simulink model "modele17"  (R2019a)
settings: Solver=VariableStepAuto  StartTime=0.0  StopTime=1  RelTol=1e-4
values from neighbouring files (symbols this model uses):
  Cb = 9.97*(10^(-2))    (= 0.0997)    [parametres_cubli.m]
  Cw = 2.95e-5    (= 2.95e-05)    [parametres_cubli.m]
  g = 9.81    [parametres_cubli.m]
  Ib = 3.43*(10^(-3))    (= 0.00343)    [parametres_cubli.m]
  Iw = 2.63*(10^(-4))    (= 0.000263)    [parametres_cubli.m]
  l = 9.65*0.01    (= 0.0965)    [parametres_cubli.m]
  lb = 10.35*0.01    (= 0.1035)    [parametres_cubli.m]
  mb = 0.43    [parametres_cubli.m]
  mw = 0.096    [parametres_cubli.m]
  Theta_b_ini = 0.125    [parametres_cubli.m]
  Tm_sat = 3.0    (= 3)    [parametres_cubli.m]
undefined symbols (not defined in the file or in its folder): K3, sigbuilder_block
settings Model: Creator=ntest557  LastModifiedBy=ntest
settings SolverCC: ZeroCrossAlgorithm=Adaptive
settings DataIOCC: ReturnWorkspaceOutputs=off
settings DebuggingCC: IgnoredZcDiagnostic=none  ArithmeticOperatorsInVariantConditions=warning
settings CodeAppCC: StateflowObjectComments=on

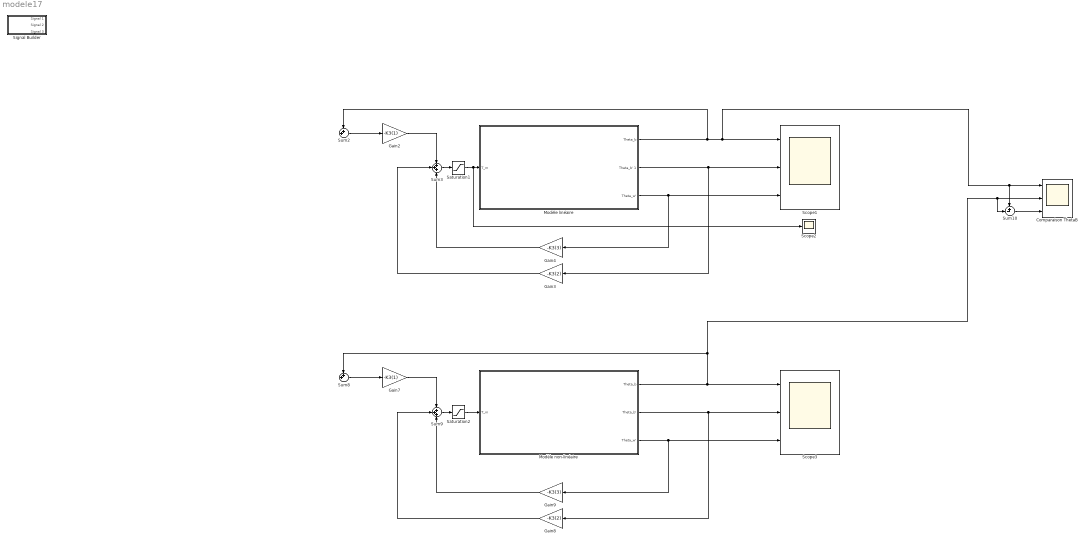
== system modele17 ==
  "Comparaison ThetaB " : Scope  NumInputPorts=3
  Gain2 : Gain  Gain=-K3(1)
  Gain3 : Gain  Gain=-K3(2)
  Gain4 : Gain  Gain=-K3(3)
  Gain7 : Gain  Gain=-K3(1)
  Gain8 : Gain  Gain=-K3(2)
  Gain9 : Gain  Gain=-K3(3)
  Modèle linéaire : Subsystem
  "Modèle non-linéaire " : Subsystem
  Saturation1 : Saturate  UpperLimit=Tm_sat  LowerLimit=-Tm_sat
  Saturation2 : Saturate  UpperLimit=Tm_sat  LowerLimit=-Tm_sat
  Scope1 : Scope  NumInputPorts=3
  Scope2 : Scope
  Scope3 : Scope  NumInputPorts=3
  Signal Builder : Subsystem  Tag=STV Subsys  LoadFcn=sigbuilder_block('load');  StartFcn=sigbuilder_block('start');  StopFcn=sigbuilder_block('stop');  ClipboardFcn=sigbuilder_block('clipboard');  mask(Sigbuilder block){tuvar=[0:10]}
      mask help: Simulink:masks:SigbuilderBlock_MD
      mask init:
      | if ~strcmp(get_param(bdroot(gcbh),'SimulationStatus'),'stopped') tuvar = sigbuilder_block('maskInit'); end
      settings: CopyFcn=sigbuilder_block('copy');  DeleteFcn=sigbuilder_block('delete');  ModelCloseFcn=sigbuilder_block('modelClose');  PreSaveFcn=sigbuilder_block('preSave');  PauseFcn=sigbuilder_block('pause');  ContinueFcn=sigbuilder_block('continue');  NameChangeFcn=sigbuilder_block('namechange');  OpenFcn=sigbuilder_block('open',[6 30 1248 660 ]);  CloseFcn=sigbuilder_block('close');
      mask Display: plot(0, 0, 100, 100,[2, 2, 32, 32, 2], [68, 8, 8, 68, 68],[32, 2], [38, 38], [32, 19, 2],[53, 60, 44], [32, 17, 17, 2],[16, 16, 31, 31]);txt = getActiveGroup(gcbh);text(2, 100, txt,'verticalAlignment', 'top');
  Sum10 : Sum  Inputs=+-|
  Sum2 : Sum  Inputs=++|
  Sum3 : Sum  Inputs=+++
  Sum8 : Sum  Inputs=++|
  Sum9 : Sum  Inputs=+++
  wires:
  "Modèle non-linéaire "/1("Theta_b ") -> Scope3/1, Sum10/2, "Comparaison ThetaB "/2, Sum8/1
  "Modèle non-linéaire "/2("Theta_b' ") -> Scope3/2, Gain8/1
  "Modèle non-linéaire "/3(Theta_w') -> Scope3/3, Gain9/1
  Sum8/1 -> Gain7/1
  Gain7/1 -> Sum9/1
  Gain8/1 -> Sum9/2
  Gain9/1 -> Sum9/3
  Sum10/1 -> "Comparaison ThetaB "/3
  Gain4/1 -> Sum3/3
  Gain3/1 -> Sum3/2
  Sum2/1 -> Gain2/1
  Gain2/1 -> Sum3/1
  Modèle linéaire/3(Theta_w') -> Scope1/3, Gain4/1
  Saturation1/1 -> Modèle linéaire/1("T_m "), Scope2/1
  Modèle linéaire/1("Theta_b ") -> Sum2/1, Sum10/1, "Comparaison ThetaB "/1, Scope1/1
  Modèle linéaire/2(Theta_b' 1) -> Gain3/1, Scope1/2
  Sum3/1 -> Saturation1/1
  Sum9/1 -> Saturation2/1
  Saturation2/1 -> "Modèle non-linéaire "/1("T_m ")

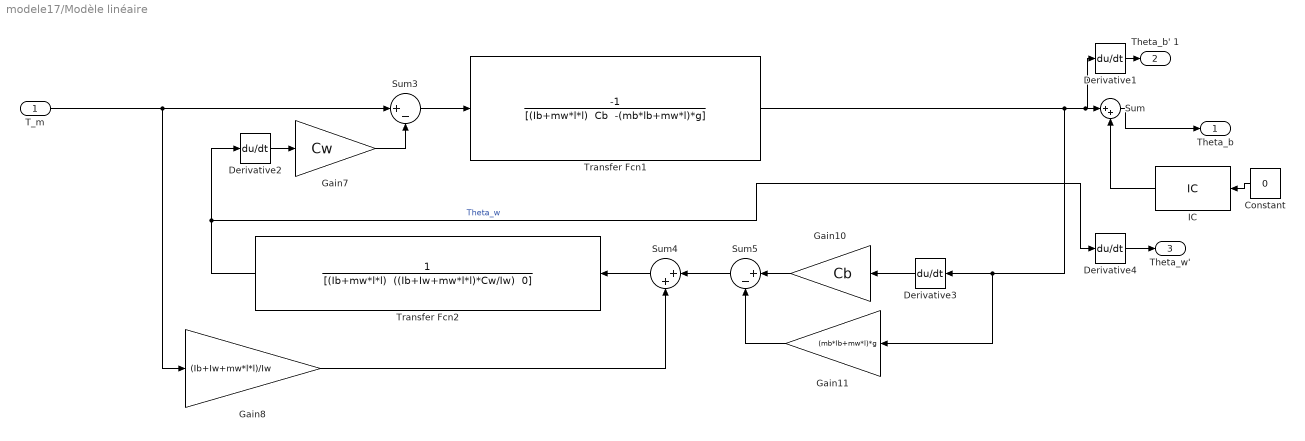
== system modele17/Modèle linéaire ==
  "T_m " : Inport
  Constant : Constant  Value=0
  Derivative{1..4} (4 alike) : Derivative
  Gain10 : Gain  Gain=Cb
  Gain11 : Gain  Gain=(mb*lb+mw*l)*g
  Gain7 : Gain  Gain=Cw
  Gain8 : Gain  Gain=(Ib+Iw+mw*l*l)/Iw
  IC : InitialCondition  Value=Theta_b_ini
  Sum : Sum  Inputs=|++
  Sum3 : Sum  Inputs=|+-
  Sum4 : Sum  Inputs=|++
  Sum5 : Sum  Inputs=|+-
  Transfer Fcn1 : TransferFcn  Numerator=[-1]  Denominator="[(Ib+mw*l*l)  Cb  -(mb*lb+mw*l)*g]"  ContinuousStateAttributes="\"Theta_b_ini\""
  Transfer Fcn2 : TransferFcn  Denominator="[(Ib+mw*l*l)  ((Ib+Iw+mw*l*l)*Cw/Iw)  0]"
  "Theta_b " : Outport
  Theta_b' 1 : Outport  Port=2
  Theta_w' : Outport  Port=3
  wires:
  Transfer Fcn2/1 -> Derivative4/1, Derivative2/1  "Theta_w"
  Gain8/1 -> Sum4/2
  Sum4/1 -> Transfer Fcn2/1
  "T_m "/1 -> Gain8/1, Sum3/1
  Gain10/1 -> Sum5/1
  Derivative2/1 -> Gain7/1
  Sum3/1 -> Transfer Fcn1/1
  Gain7/1 -> Sum3/2
  Derivative3/1 -> Gain10/1
  Sum5/1 -> Sum4/1
  Gain11/1 -> Sum5/2
  Derivative4/1 -> Theta_w'/1
  Derivative1/1 -> Theta_b' 1/1
  Transfer Fcn1/1 -> Derivative3/1, Gain11/1, Derivative1/1, Sum/1
  Sum/1 -> "Theta_b "/1
  Constant/1 -> IC/1
  IC/1 -> Sum/2

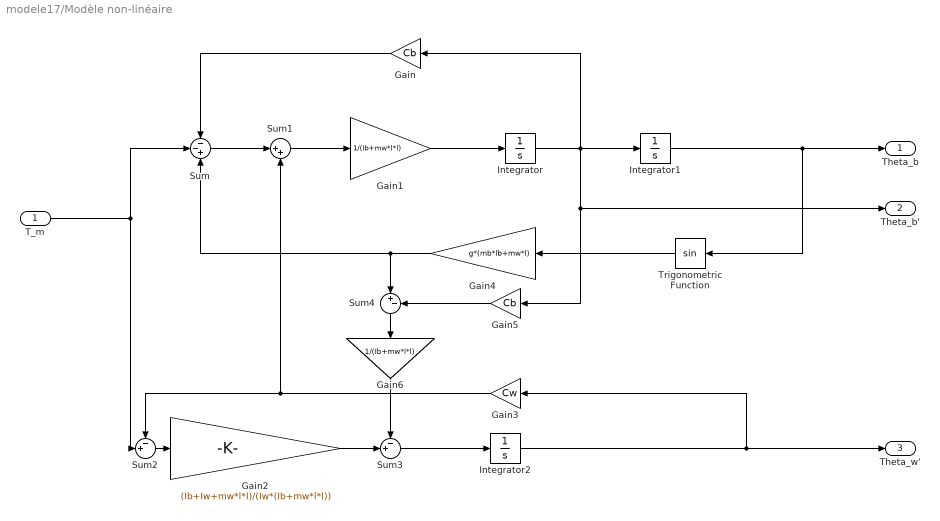
== system modele17/Modèle non-linéaire  ==
  "T_m " : Inport
  Gain : Gain  Gain=Cb
  Gain1 : Gain  Gain=1/(Ib+mw*l*l)
  Gain2 : Gain  Gain=(Ib+Iw+mw*l*l)/(Iw*(Ib+mw*l*l))
  Gain3 : Gain  Gain=Cw
  Gain4 : Gain  Gain=g*(mb*lb+mw*l)
  Gain5 : Gain  Gain=Cb
  Gain6 : Gain  Gain=1/(Ib+mw*l*l)
  Integrator : Integrator
  Integrator1 : Integrator  InitialCondition=Theta_b_ini
  Integrator2 : Integrator
  Sum : Sum  Inputs=--+
  Sum1 : Sum  Inputs=|++
  Sum2 : Sum  Inputs=-+|
  Sum3 : Sum  Inputs=-+|
  Sum4 : Sum  Inputs=|+-
  Trigonometric Function : Trigonometry
  "Theta_b " : Outport
  "Theta_b' " : Outport  Port=2
  Theta_w' : Outport  Port=3
  wires:
  Gain/1 -> Sum/1
  Sum/1 -> Sum1/1
  Sum1/1 -> Gain1/1
  Gain1/1 -> Integrator/1
  Integrator/1 -> "Theta_b' "/1, Gain5/1, Gain/1, Integrator1/1
  "T_m "/1 -> Sum/2, Sum2/2
  Integrator1/1 -> Trigonometric Function/1, "Theta_b "/1
  Sum2/1 -> Gain2/1
  Gain2/1 -> Sum3/2
  Sum3/1 -> Integrator2/1
  Integrator2/1 -> Gain3/1, Theta_w'/1
  Gain3/1 -> Sum1/2, Sum2/1
  Trigonometric Function/1 -> Gain4/1
  Gain4/1 -> Sum/3, Sum4/1
  Sum4/1 -> Gain6/1
  Gain5/1 -> Sum4/2
  Gain6/1 -> Sum3/1

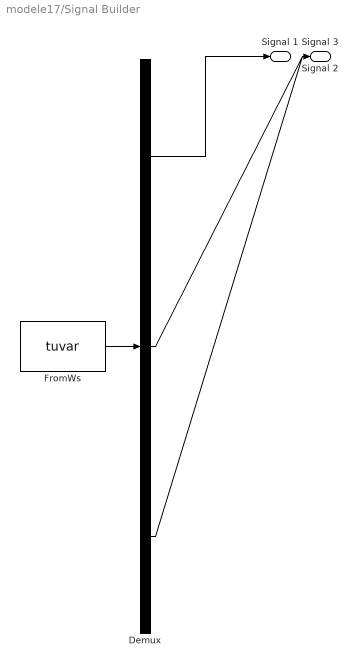
== system modele17/Signal Builder ==
  Demux : Demux  Tag=STV Demux  Outputs=3
  FromWs : FromWorkspace  Tag=STV FromWs  VariableName=tuvar  SampleTime=0
      SigBuilderData=|
      | common.afterFinalStr = 'Extrapolate'
      | common.sampleTime = 0
      | dataSet.timeRange = [0 10]
      | dataSet.name = 'Group 1'
      | sbobj.Groups.Name = 'Group 1'
      | sbobj.Groups.Signals(1).Name = 'Signal 1'
      | sbobj.Groups.Signals(1).XData = [0 3.98 3.98 4.48 4.48 4.98 4.98 5.48 5.48 9.98 10]
      | sbobj.Groups.Signals(1).YData = [0 0 0.1 0.1 0 0 -0.1 -0.1 0 0 0]
      | sbobj.Groups.Signals(2).Name = 'Signal 2'
      | sbobj.Groups.Signals(2).XData = [0 4 5 10]
      | sbobj.Groups.Signals(2).YData = [0 0 0.01 0.01]
      | sbobj.Groups.Signals(3).Name = 'Signal 3'
      | sbobj.Groups.Signals(3).XData = [0 0.1 0.1 2 6 10]
      | sbobj.Groups.Signals(3).YData = [0.2 0.2 0 0 0 0]
  Signal 1 : Outport  Tag=STV Outport
  Signal 2 : Outport  Tag=STV Outport  Port=2
  Signal 3 : Outport  Tag=STV Outport  Port=3
  wires:
  Demux/1 -> Signal 1/1
  FromWs/1 -> Demux/1
  Demux/2 -> Signal 2/1
  Demux/3 -> Signal 3/1
